simulink model "pentek_dac_ip_test"  (R2019b)
settings: Solver=FixedStepDiscrete  StartTime=0.0  StopTime=10e-6  FixedStep=fpga_Ts  RelTol=1e-3
PreLoadFcn:
  | model_init;
InitFcn:
  | model_init;
values from neighbouring files (symbols this model uses):
  Fs = ConverterSamplingRate/DDC_DUC_factor    (= 2000000000)    [model_init.m]
  NCO_WL = 16    [model_init.m]
  VectorSamplingFactor = 4    [model_init.m]
undefined symbols (not defined in the file or in its folder): Fo
libraries: dsphdlsigops x1
settings Model: DataTypeOverride=Off  Creator=tmealey  LastModifiedBy=larry
settings DataIOCC: SignalLogging=off  DSMLogging=off  ReturnWorkspaceOutputs=off
settings OptimizationCC: BlockReduction=off  ConditionallyExecuteInputs=off  DefaultParameterBehavior=Inlined
settings DebuggingCC: AlgebraicLoopMsg=error  SingleTaskRateTransMsg=error
settings HardwareCC: ProdBitPerPointer=32  ProdBitPerSizeT=32  ProdBitPerPtrDiffT=32  ProdLargestAtomicFloat=None  ProdIntDivRoundTo=Undefined  ProdEndianess=Unspecified  ProdWordSize=32  ProdHWDeviceType=ASIC/FPGA->ASIC/FPGA  TargetBitPerPointer=64  TargetBitPerSizeT=64  TargetBitPerPtrDiffT=64  TargetLongLongMode=on  TargetIntDivRoundTo=Zero  TargetEndianess=LittleEndian  TargetWordSize=64  TargetHWDeviceType=Custom Processor->MATLAB Host Computer  ProdEqTarget=off

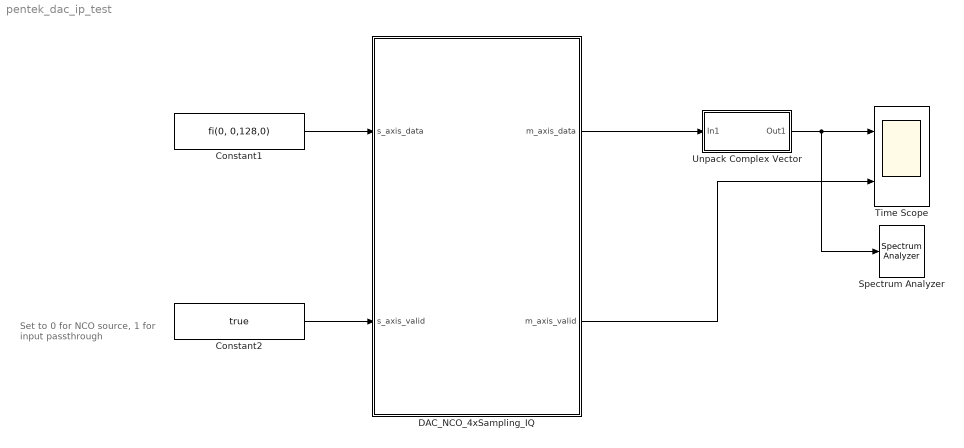
== system pentek_dac_ip_test ==
  note: Set to 0 for NCO source,
      | 1 for input passthrough
  Constant1 : Constant  Value=fi(0, 0,128,0)  SampleTime=-1
  Constant2 : Constant  Value=true  SampleTime=-1
  DAC_NCO_4xSampling_IQ : Subsystem  TreatAsAtomicUnit=on
  Spectrum Analyzer : SpectrumAnalyzer
  Time Scope : Scope  NumInputPorts=2
  Unpack Complex Vector : Subsystem  mask(Convert packed word to complex vector.){datatype=fixdt(1,16,15), VectorLength=VectorSamplingFactor}
      mask prompts: datatype "Output datatype:"; VectorLength "Vector length:"
      mask help: Input word has real and imaginary components interleaved, with the first real vector element in the LSB and the last imaginary element in the MSB.
      mask init:
      | OutputWordLength = numerictype(datatype).WordLength;
      | 
      | Simulink.suppressDiagnostic(gcbh,...
      |  'SimulinkFixedPoint:util:Overflowoccurred');
      mask Display: fprintf('Unpack\nComplex\nVector');
  wires:
  Constant1/1 -> DAC_NCO_4xSampling_IQ/1(s_axis_data)
  Constant2/1 -> DAC_NCO_4xSampling_IQ/2(s_axis_valid)
  DAC_NCO_4xSampling_IQ/2(m_axis_valid) -> Time Scope/2
  DAC_NCO_4xSampling_IQ/1(m_axis_data) -> Unpack Complex Vector/1(In1)
  Unpack Complex Vector/1(Out1) -> Spectrum Analyzer/1, Time Scope/1

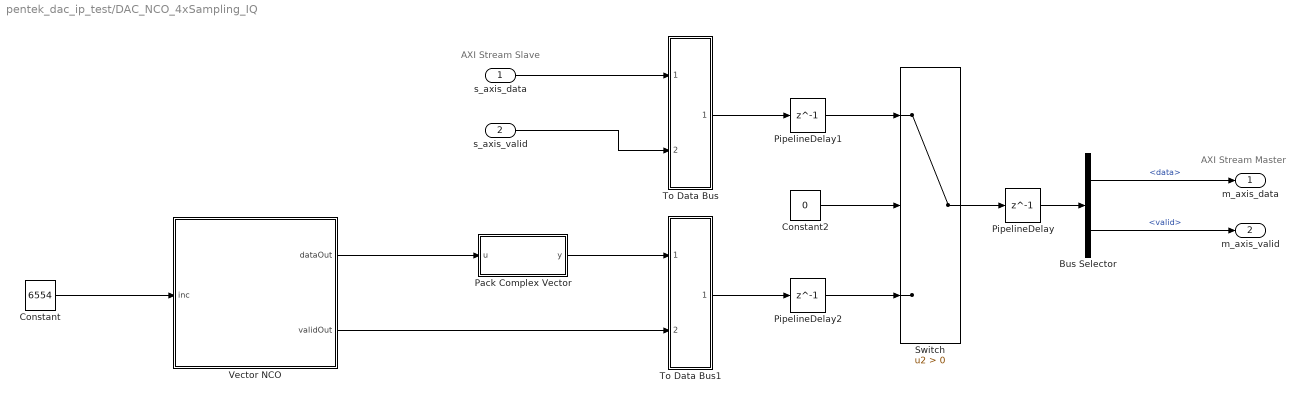
== system pentek_dac_ip_test/DAC_NCO_4xSampling_IQ ==
  note: AXI Stream Slave
  note: AXI Stream Master
  s_axis_data : Inport
  s_axis_valid : Inport  Port=2
  Bus Selector : BusSelector  OutputSignals=data,valid
  Constant : Constant  Value=6554  OutDataTypeStr=uint32  SampleTime=-1
  Constant2 : Constant  Value=0  OutDataTypeStr=fixdt(0,1)  SampleTime=-1
  Pack Complex Vector : Subsystem  mask(Pack Complex Vector){}
      mask help:
      | Convert complex vector to packed word.
      |
      | Real and imaginary components are interleaved, with real component starting in LSB position.
      |
      | The first vector element is placed in the LSB, and the last vector element is placed in the MSB.
      mask Display: fprintf('Pack\nComplex\nVector');
  PipelineDelay : Delay  DelayLength=1
  PipelineDelay1 : Delay  DelayLength=1
  PipelineDelay2 : Delay  DelayLength=1
  Switch : Switch  Criteria=u2 > Threshold
  To Data Bus : Subsystem
  To Data Bus1 : Subsystem
  Vector NCO : Subsystem  mask{N=NCO_WL, factor=4, OUT_WL=NCO_WL, OUT_FL=NCO_WL-1}
      mask prompts: N "Accumulator word length:"; factor "Vectorization factor:"; OUT_WL "Output word length:"; OUT_FL "Output fraction length:"
      mask init:
      | offsetIdx = 0:(factor-1);
  m_axis_data : Outport
  m_axis_valid : Outport  Port=2
  wires:
  Constant/1 -> Vector NCO/1(inc)
  Vector NCO/1(dataOut) -> Pack Complex Vector/1(u)
  Pack Complex Vector/1(y) -> To Data Bus1/1(data)
  s_axis_data/1 -> To Data Bus/1(data)
  s_axis_valid/1 -> To Data Bus/2(valid)
  Vector NCO/2(validOut) -> To Data Bus1/2(valid)
  To Data Bus1/1(bus) -> PipelineDelay2/1
  Constant2/1 -> Switch/2
  To Data Bus/1(bus) -> PipelineDelay1/1
  Switch/1 -> PipelineDelay/1
  Bus Selector/1 -> m_axis_data/1  "<data>"
  Bus Selector/2 -> m_axis_valid/1  "<valid>"
  PipelineDelay/1 -> Bus Selector/1
  PipelineDelay1/1 -> Switch/1
  PipelineDelay2/1 -> Switch/3

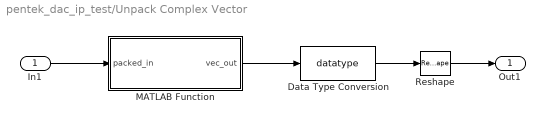
== system pentek_dac_ip_test/Unpack Complex Vector ==
  In1 : Inport
  Data Type Conversion : DataTypeConversion  OutDataTypeStr=datatype  ConvertRealWorld=Stored Integer (SI)
  MATLAB Function : MATLAB Function  TreatAsAtomicUnit=on
  Reshape : Reshape  OutputDimensionality=Column vector (2-D)
  Out1 : Outport  VectorParamsAs1DForOutWhenUnconnected=off
  wires:
  Data Type Conversion/1 -> Reshape/1
  In1/1 -> MATLAB Function/1(packed_in)
  MATLAB Function/1(vec_out) -> Data Type Conversion/1
  Reshape/1 -> Out1/1

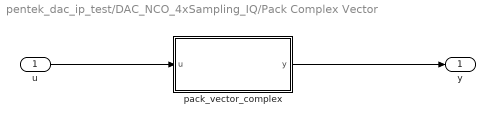
== system pentek_dac_ip_test/DAC_NCO_4xSampling_IQ/Pack Complex Vector ==
  u : Inport
  pack_vector_complex : MATLAB Function  TreatAsAtomicUnit=on
  y : Outport
  wires:
  u/1 -> pack_vector_complex/1(u)
  pack_vector_complex/1(y) -> y/1

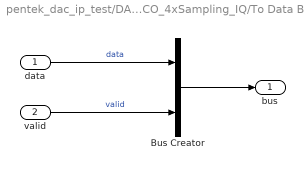
== system pentek_dac_ip_test/DAC_NCO_4xSampling_IQ/To Data Bus ==
  data : Inport
  valid : Inport  Port=2
  Bus Creator : BusCreator  Inputs=2
  bus : Outport
  wires:
  Bus Creator/1 -> bus/1
  valid/1 -> Bus Creator/2  "valid"
  data/1 -> Bus Creator/1  "data"

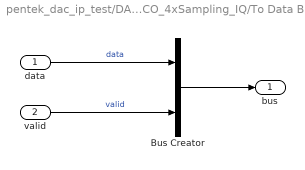
== system pentek_dac_ip_test/DAC_NCO_4xSampling_IQ/To Data Bus1 ==
  data : Inport
  valid : Inport  Port=2
  Bus Creator : BusCreator  Inputs=2
  bus : Outport
  wires:
  data/1 -> Bus Creator/1  "data"
  valid/1 -> Bus Creator/2  "valid"
  Bus Creator/1 -> bus/1

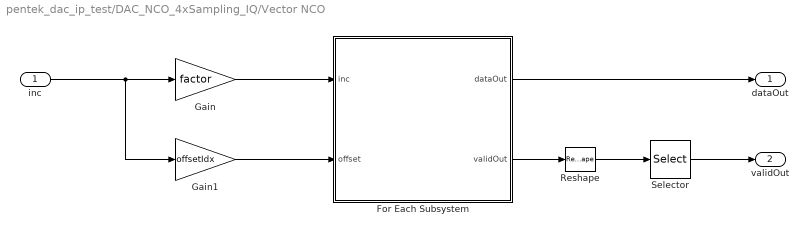
== system pentek_dac_ip_test/DAC_NCO_4xSampling_IQ/Vector NCO ==
  inc : Inport
  For Each Subsystem : Subsystem  TreatAsAtomicUnit=on
  Gain : Gain  Gain=factor  OutDataTypeStr=Inherit: Same as input  ParamDataTypeStr=Inherit: Same as input
  Gain1 : Gain  Gain=offsetIdx  OutDataTypeStr=Inherit: Same as input  ParamDataTypeStr=Inherit: Same as input
  Reshape : Reshape
  Selector : Selector  InputPortWidth=factor  IndexOptions=Index vector (dialog)  Indices=1  OutputSizes=1
  dataOut : Outport
  validOut : Outport  Port=2
  wires:
  inc/1 -> Gain1/1, Gain/1
  For Each Subsystem/2(validOut) -> Reshape/1
  Selector/1 -> validOut/1
  Reshape/1 -> Selector/1
  For Each Subsystem/1(dataOut) -> dataOut/1
  Gain/1 -> For Each Subsystem/1(inc)
  Gain1/1 -> For Each Subsystem/2(offset)

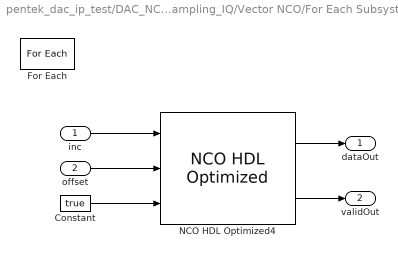
== system pentek_dac_ip_test/DAC_NCO_4xSampling_IQ/Vector NCO/For Each Subsystem ==
  inc : Inport
  offset : Inport  Port=2  Partition=on  PartitionDimension=1  PartitionWidth=1  PartitionOffset=0
  Constant : Constant  Value=true  SampleTime=-1
  For Each : ForEach  DisableCoverage=on
  NCO HDL Optimized4 : dsphdlsigops/NCO HDL Optimized  PhaseIncrementSource=Input port  PhaseIncrement=round(Fo*(2^N)/Fs)  PhaseOffsetSource=Input port  PhaseOffset=0  DitherSource=None  NumDitherBits=4  PhaseQuantization=off  NumQuantizerAccumulatorBits=12  LUTCompress=on  ResetAction=off  ValidInputPort=on  Waveform=Complex exponential  PhasePort=off  SimulateUsing=Code generation  AccumulatorWL=N  OutputDataType=Binary point scaling  OutputWL=OUT_WL  OutputFL=OUT_FL
      settings: SourceProductBaseCode=DS
  dataOut : Outport  ConcatenationDimension=1
  validOut : Outport  Port=2  ConcatenationDimension=1
  wires:
  NCO HDL Optimized4/1 -> dataOut/1
  inc/1 -> NCO HDL Optimized4/1
  NCO HDL Optimized4/2 -> validOut/1
  offset/1 -> NCO HDL Optimized4/2
  Constant/1 -> NCO HDL Optimized4/3

== matlab function pentek_dac_ip_test/DAC_NCO_4xSampling_IQ/Pack Complex Vector/pack_vector_complex ==
  data: u input; y output
function y = pack_vector_complex(u)
%#codegen

assert(~isreal(u),'Expected input to be complex');

N = coder.const(numel(u));

temp = coder.nullcopy((cast_to_fi(zeros([N*2 1],'like',real(u)))));

% Interleave real/imag
coder.unroll();
for ii=N:-1:1
    temp((ii-1)*2+2) = real(u(N-ii+1));
    temp((ii-1)*2+1) = imag(u(N-ii+1));
end

y = bitconcat(temp);

== matlab function pentek_dac_ip_test/Unpack Complex Vector/MATLAB Function ==
  data: packed_in input; vec_out output; OutputWordLength parameter; VectorLength parameter
function vec_out = unpack_complex_vector(packed_in, OutputWordLength, VectorLength)
%#codegen

OUT_WL = coder.const(OutputWordLength);
NUM_WORDS = coder.const(VectorLength);

packed_in_fi = cast_to_fi(packed_in);

temp = coder.nullcopy(fi(complex(zeros(NUM_WORDS,1)), 0,OUT_WL,0));
coder.unroll();
for ii=1:NUM_WORDS
   temp(ii) = complex(...
       bitsliceget(packed_in_fi, (ii-1)*2*OUT_WL + OUT_WL, (ii-1)*2*OUT_WL + 1), ...
       bitsliceget(packed_in_fi, (ii*2-1)*OUT_WL + OUT_WL, (ii*2-1)*OUT_WL + 1));
end

vec_out = temp;
